simulink model "simulinkcorregidoquartercar2"  (R2020b)
settings: Solver=VariableStepAuto  StartTime=0.0  StopTime=10  RelTol=1e-3
values from neighbouring files (symbols this model uses):
  Gr = 2.56e-6    (= 2.56e-06)    [custom_mainNORMAL.m]
  vcar = vcar_arra(idxcar)/3.6    [custom_mainNORMAL.m]
  wcut = 2*pi*vcar/100    [custom_mainNORMAL.m]
undefined symbols (not defined in the file or in its folder): SS
libraries: simulink x1, slctrlblks x1
settings Model: Creator=Slayer  LastModifiedBy=kevin
settings SFSimCC: CustomCodeUndefinedFunction=UseInterfaceOnly

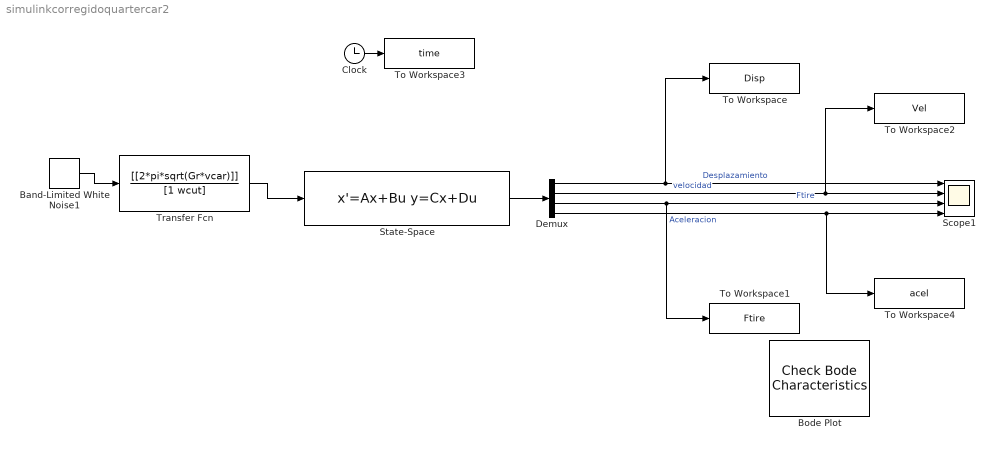
== system simulinkcorregidoquartercar2 ==
  Band-Limited White Noise1 : simulink/Sources/Band-Limited White Noise  Cov=[0.5]  Ts=0.001  seed=[23341]
  Bode Plot : slctrlblks/Model Verification/Check Bode  Characteristics  InstantiateOnLoad=on  SaveOperatingPoints=off  LinearizationIOs={'/Transfer Fcn', 1, 'in', 'off', '';'/Demux', 3, 'out', 'on', ''}  LinearizeAt=SnapshotTimes  SnapshotTimes=[0]  TriggerType=rising  SampleTime=auto  RateConversionMethod=zoh  PreWarpFreq=10  UseExactDelayModel=off  UseFullBlockNameLabels=off  UseBusSignalLabels=off  enabled=on  stopWhenAssertionFail=off  export=off  ViewDlgPos=[1 1121 1280 683]  OpenViewOnLoad=off  LaunchViewOnOpen=on  FrequencyUnits=rad/s  MagnitudeUnits=dB  PhaseUnits=deg  TimeUnits=seconds  EnableUpperBound=off  UpperBoundFrequencies=[]  UpperBoundMagnitudes=[]  EnableLowerBound=off  LowerBoundFrequencies=[]  LowerBoundMagnitudes=[]
      settings: SaveToWorkspace=on  SaveName=passive
  Clock : Clock
  Demux : Demux
  Scope1 : Scope  NumInputPorts=4
  State-Space : StateSpace  A=SS.A  B=SS.B  C=SS.C  D=SS.D  InitialCondition=0
  To Workspace : ToWorkspace  VariableName=Disp  SampleTime=0.001
  To Workspace1 : ToWorkspace  VariableName=Ftire  SampleTime=0.001
  To Workspace2 : ToWorkspace  VariableName=Vel  SampleTime=0.001
  To Workspace3 : ToWorkspace  VariableName=time  SampleTime=0.001
  To Workspace4 : ToWorkspace  VariableName=acel  SampleTime=0.001
  Transfer Fcn : TransferFcn  Numerator=[[2*pi*sqrt(Gr*vcar)]]  Denominator=[1 wcut]
  wires:
  Demux/2 -> To Workspace2/1, Scope1/2  "velocidad"
  State-Space/1 -> Demux/1
  Demux/1 -> To Workspace/1, Scope1/1  "Desplazamiento"
  Demux/3 -> Scope1/3, To Workspace1/1  "Ftire"
  Clock/1 -> To Workspace3/1
  Demux/4 -> Scope1/4, To Workspace4/1  "Aceleracion"
  Transfer Fcn/1 -> State-Space/1
  Band-Limited White Noise1/1 -> Transfer Fcn/1
